simulink model "modle_test"  (R2016a)
settings: Solver=VariableStepAuto  StartTime=0.0  StopTime=5  RelTol=1e-3
libraries: simulink x1
settings Model: Creator=Shinelon  LastModifiedBy=Shinelon

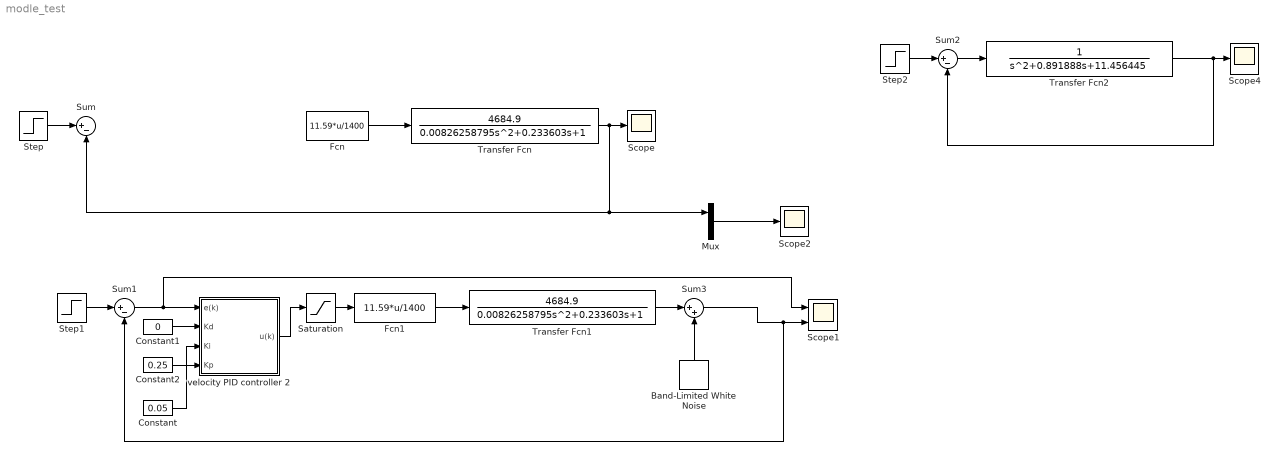
== system modle_test ==
  Band-Limited White Noise : simulink/Sources/Band-Limited White Noise  Cov=1  Ts=0.005  seed=[23341]
  Constant : Constant  Value=0.05  OutMax=[1400]
  Constant1 : Constant  Value=0  OutMax=[1400]
  Constant2 : Constant  Value=0.25  OutMax=[1400]
  Fcn : Fcn  Expr=11.59*u/1400
  Fcn1 : Fcn  Expr=11.59*u/1400
  Mux : Mux  Inputs=2
  Saturation : Saturate  UpperLimit=1400  LowerLimit=-1400
  Scope : Scope
  Scope1 : Scope  NumInputPorts=2
  Scope2 : Scope
  Scope4 : Scope
  Step : Step  Time=0.11  After=9000  SampleTime=0.005
  Step1 : Step  Time=0  After=2000  SampleTime=0.005
  Step2 : Step  Time=0  SampleTime=0.005
  Sum : Sum  Inputs=|+-
  Sum1 : Sum  Inputs=|+-
  Sum2 : Sum  Inputs=|+-
  Sum3 : Sum  Inputs=|++
  Transfer Fcn : TransferFcn  Numerator=[4684.9]  Denominator="[0.00826258795  0.233603 1]"
  Transfer Fcn1 : TransferFcn  Numerator=[4684.9]  Denominator="[0.00826258795  0.233603 1]"
  Transfer Fcn2 : TransferFcn  Denominator="[1  0.891888 11.456445]"
  velocity PID controller 2 : Subsystem
  wires:
  Transfer Fcn/1 -> Sum/2, Mux/1, Scope/1
  Step/1 -> Sum/1
  Step1/1 -> Sum1/1
  Sum1/1 -> Scope1/1, velocity PID controller 2/1(e(k))
  Constant/1 -> velocity PID controller 2/4("Kp ")
  Constant1/1 -> velocity PID controller 2/2("Kd ")
  Constant2/1 -> velocity PID controller 2/3("Ki ")
  Mux/1 -> Scope2/1
  Fcn/1 -> Transfer Fcn/1
  Fcn1/1 -> Transfer Fcn1/1
  Transfer Fcn2/1 -> Scope4/1, Sum2/2
  Step2/1 -> Sum2/1
  Sum2/1 -> Transfer Fcn2/1
  Saturation/1 -> Fcn1/1
  velocity PID controller 2/1(u(k)) -> Saturation/1
  Transfer Fcn1/1 -> Sum3/1
  Sum3/1 -> Scope1/2, Sum1/2
  Band-Limited White Noise/1 -> Sum3/2

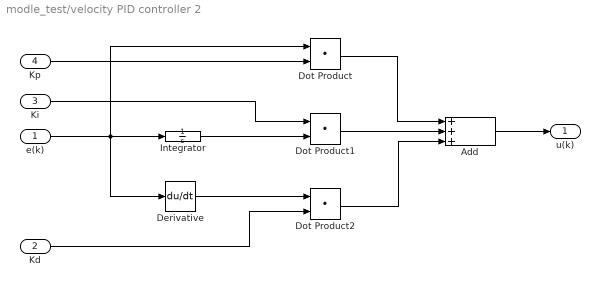
== system modle_test/velocity PID controller 2 ==
  e(k) : Inport
  "Kd " : Inport  Port=2
  "Ki " : Inport  Port=3
  "Kp " : Inport  Port=4
  Add : Sum  Inputs=+++
  Derivative : Derivative
  Dot Product : DotProduct  InputSameDT=on  OutDataTypeStr=Inherit: Inherit via internal rule
  Dot Product1 : DotProduct  InputSameDT=on  OutDataTypeStr=Inherit: Inherit via internal rule
  Dot Product2 : DotProduct  InputSameDT=on  OutDataTypeStr=Inherit: Inherit via internal rule
  Integrator : Integrator
  u(k) : Outport
  wires:
  e(k)/1 -> Derivative/1, Integrator/1, Dot Product/1
  Dot Product1/1 -> Add/2
  "Kd "/1 -> Dot Product2/2
  Integrator/1 -> Dot Product1/2
  Dot Product2/1 -> Add/3
  Dot Product/1 -> Add/1
  Derivative/1 -> Dot Product2/1
  Add/1 -> u(k)/1
  "Kp "/1 -> Dot Product/2
  "Ki "/1 -> Dot Product1/1
